simulink model "dvb_s2_channel"  (R2025b)
settings: Solver=VariableStepAuto  StartTime=0.0  StopTime=1  RelTol=1e-3
undefined symbols (not defined in the file or in its folder): RRC_reseive, Ts
libraries: dspsrcs4 x5, commfilt2 x2, commchan3 x1, whdlmod x1, commsync2 x1
settings Model: Creator=Пётр  LastModifiedBy=Пётр

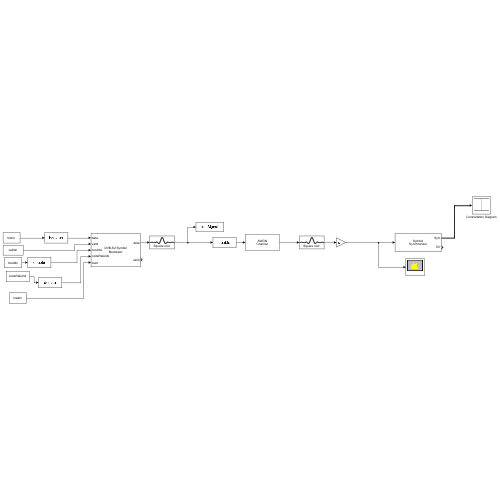
[thumbnail: Simulink's stored preview of the top-level diagram]
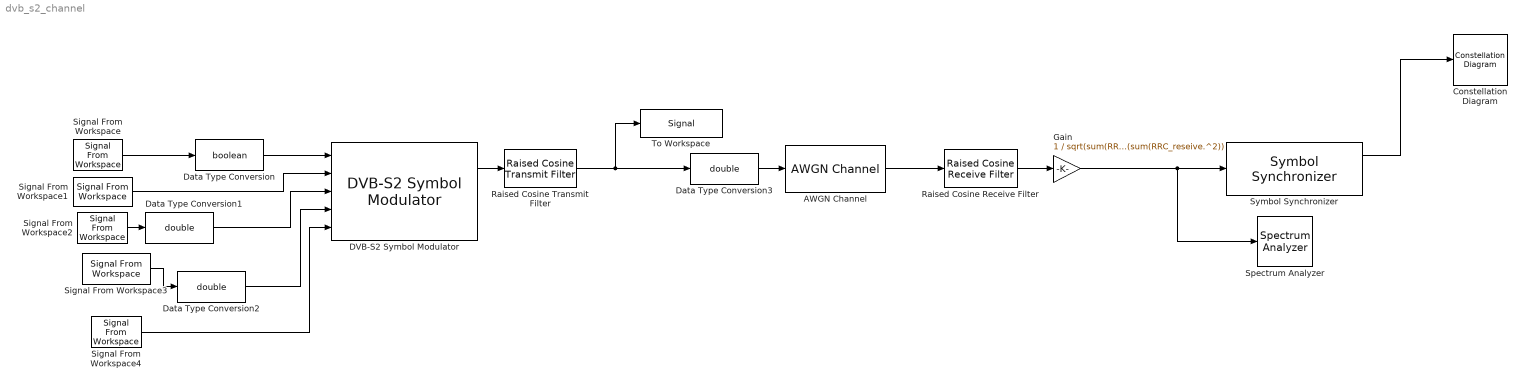
== system dvb_s2_channel ==
  AWGN Channel : commchan3/AWGN Channel  LegacyMode=off  NoiseMethod="Signal to noise ratio  (SNR)"  noiseMode="Signal to noise ratio  (SNR)"  EbNo=10  EsNo=10  SNR=6  BitsPerSymbol=1  SignalPower=1  SpecifySymbolPeriod=off  SamplesPerSymbol=1  SymbolPeriod=1  VarianceSource=Parameter  Variance=1  RandomStream=Global stream  Seed=67  SimulateUsing=Code generation
  Constellation Diagram : ConstellationDiagram  WindowPosition=[925.000000,305.000000,282.000000,294.000000,]  ScopeFrameLocation=window  SymbolsToDisplaySource=Property  SymbolsToDisplay=1000  ReferenceConstellation="[0.70711+0.70711i        -0.70711+0.70711i        -0.70711-0.70711i         0.70711-0.70711i]"  ShowLegend=on  MeasurementInterval=1000
  DVB-S2 Symbol Modulator : whdlmod/DVB-S2 Symbol Modulator  ModulationSourceParams=Input port  ModulationScheme=QPSK  CodeRateAPSK=3/4  UnitAveragePower=on  SimulateUsing=Code generation  OutputDataType=Custom  WordLength=16
  Data Type Conversion : DataTypeConversion  OutDataTypeStr=boolean  SaturateOnIntegerOverflow=off  RndMeth=Floor
  Data Type Conversion1 : DataTypeConversion  OutDataTypeStr=double  SaturateOnIntegerOverflow=off  RndMeth=Floor
  Data Type Conversion2 : DataTypeConversion  OutDataTypeStr=double  SaturateOnIntegerOverflow=off  RndMeth=Floor
  Data Type Conversion3 : DataTypeConversion  OutDataTypeStr=double  SaturateOnIntegerOverflow=off  RndMeth=Floor
  Gain : Gain  Gain="1 / sqrt(sum(RRC_reseive.^2)) /  sqrt(sum(RRC_reseive.^2))"
  Raised Cosine Receive Filter : commfilt2/Raised Cosine Receive Filter  filtType=Square root  R=0.25  filtSpan=10  N=8  downFactor=8  downOffset=0  filterGain=10  InputProcessing=Columns as channels (frame based)  RateOptions=Enforce single-rate processing  framing=Mute  checkCoeff=on  variableName=RRC_reseive  currentFiltSpan=10  D=5  inputOffset=0  sampMode=Mute  saveAsFlag=0  rateMode=Downsampling  checkGain=Normalized  launchFVT=on  roundingMode=Floor  overflowMode=off  coeffDataTypeStr=Inherit: Same word length as input  coeffMin=[]  coeffMax=[]  coeffLastDataTypeStr=Inherit: Same word length as input  accumDataTypeStr=Inherit: Same as product output  accumLastDataTypeStr=Inherit: Same as product output  outputDataTypeStr=Inherit: Same as accumulator  outputMin=[]  outputMax=[]  outputLastDataTypeStr=Inherit: Same as accumulator
  Raised Cosine Transmit Filter : commfilt2/Raised Cosine Transmit Filter  filtType=Square root  R=0.25  filtSpan=10  N=8  filterGain=10  InputProcessing=Columns as channels (frame based)  RateOptions=Enforce single-rate processing  framing=Mute  checkCoeff=off  variableName=rcTxFilt  checkGain=Normalized  sampMode=Mute  saveAsFlag=0  currentFiltSpan=10  D=(10)/2  launchFVT=on  roundingMode=Floor  overflowMode=off  coeffDataTypeStr=Inherit: Same word length as input  coeffMin=[]  coeffMax=[]  coeffLastDataTypeStr=Inherit: Same word length as input  outputDataTypeStr=Inherit: Same as accumulator  outputMin=[]  outputMax=[]  outputLastDataTypeStr=Inherit: Same as accumulator
  Signal From Workspace : dspsrcs4/Signal From Workspace  X=bitsIn  Ts=Ts  nsamps=1  OutputAfterFinalValue=Setting to zero  ignoreOrWarnInputAndFrameLengths=off  OutputFrames=off
  Signal From Workspace1 : dspsrcs4/Signal From Workspace  X=validIn  Ts=Ts  nsamps=1  OutputAfterFinalValue=Setting to zero  ignoreOrWarnInputAndFrameLengths=off  OutputFrames=off
  Signal From Workspace2 : dspsrcs4/Signal From Workspace  X=modIdn  Ts=Ts  nsamps=1  OutputAfterFinalValue=Setting to zero  ignoreOrWarnInputAndFrameLengths=off  OutputFrames=off
  Signal From Workspace3 : dspsrcs4/Signal From Workspace  X=codeRateInd  Ts=Ts  nsamps=1  OutputAfterFinalValue=Setting to zero  ignoreOrWarnInputAndFrameLengths=off  OutputFrames=off
  Signal From Workspace4 : dspsrcs4/Signal From Workspace  X=loadIn  Ts=Ts  nsamps=1  OutputAfterFinalValue=Setting to zero  ignoreOrWarnInputAndFrameLengths=off  OutputFrames=off
  Spectrum Analyzer : SpectrumAnalyzer  WindowPosition=[226.000000,362.000000,567.000000,316.000000,]  ScopeFrameLocation=window  SampleRate=100000000  Span=1000000  StartFrequency=-500000  StopFrequency=500000  AveragingMethod=Exponential  YLimits=[-7.0369 0.1074]  ShowLegend=on  AllowFFTLengthLessThanSamplesPerUpdate=on
  Symbol Synchronizer : commsync2/Symbol Synchronizer  Modulation=PAM/PSK/QAM  TimingErrorDetector=Early-Late (non-data-aided)  SamplesPerSymbol=8  DampingFactor=1  NormalizedLoopBandwidth=0.01  DetectorGain=2.7  TimingErrorOutputPort=on  SimulateUsing=Code generation
  To Workspace : ToWorkspace  VariableName=Signal  SampleTime=Ts
      settings: Save2DSignal=2-D array (concatenate along first dimension)
  wires:
  Data Type Conversion/1 -> DVB-S2 Symbol Modulator/1
  Signal From Workspace/1 -> Data Type Conversion/1
  Signal From Workspace1/1 -> DVB-S2 Symbol Modulator/2
  Signal From Workspace4/1 -> DVB-S2 Symbol Modulator/5
  Signal From Workspace2/1 -> Data Type Conversion1/1
  Data Type Conversion1/1 -> DVB-S2 Symbol Modulator/3
  Signal From Workspace3/1 -> Data Type Conversion2/1
  Data Type Conversion2/1 -> DVB-S2 Symbol Modulator/4
  DVB-S2 Symbol Modulator/1 -> Raised Cosine Transmit Filter/1
  Raised Cosine Transmit Filter/1 -> To Workspace/1, Data Type Conversion3/1
  Data Type Conversion3/1 -> AWGN Channel/1
  AWGN Channel/1 -> Raised Cosine Receive Filter/1
  Raised Cosine Receive Filter/1 -> Gain/1
  Gain/1 -> Spectrum Analyzer/1, Symbol Synchronizer/1
  Symbol Synchronizer/1 -> Constellation Diagram/1
